simulink model "sym-project"  (R2023b)
settings: Solver=VariableStepAuto  StartTime=0.0  StopTime=5  RelTol=1e-3
undefined symbols (not defined in the file): A1_val, a1_val, A2_val, a2_val, A3_val, a3_val, A4_val, a4_val, A_numeric, B_numeric, C_numeric, g_val, K, k1, k1_val, k2_val, k_f, K_i, l_t, landa1_val, landa2_val
libraries: simulink x1
settings Model: Creator=Windows 10 2A-2017  LastModifiedBy=Asus
settings OptimizationCC: ReuseModelBlockBuffer=off

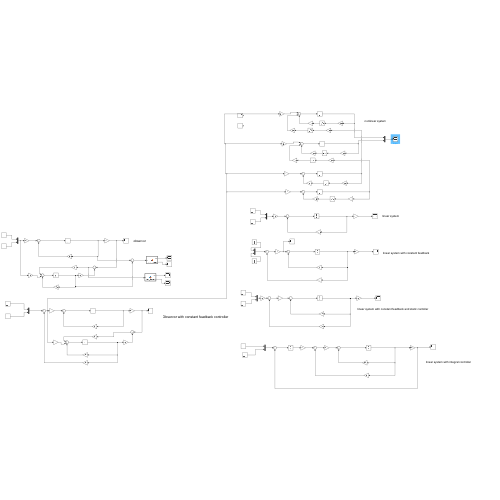
[thumbnail: Simulink's stored preview of the top-level diagram]
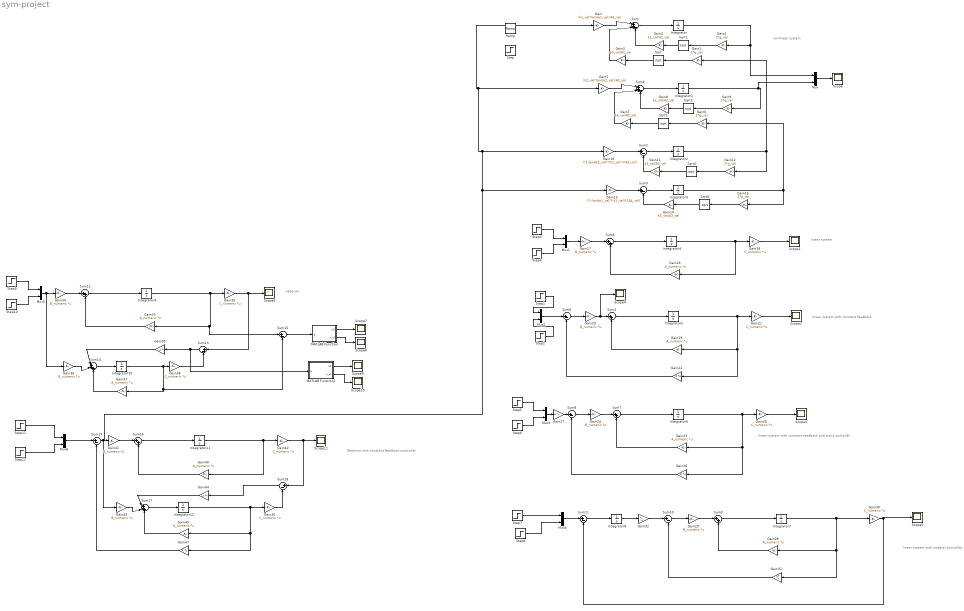
== system sym-project ==
  note: Observor with constant feadback controller
  note: linear system with constant feadback
  note: linear system
  note: nonlinear system
  note: linear system with constant feadback and static contoller
  note: linear system with integral controller
  note: observor
  Gain : Gain  Gain=(k1_val*landa1_val)/A1_val
  Gain{1,4,6,9,12,15} (6 alike) : Gain  Gain=2*g_val
  Gain10 : Gain  Gain=((1-landa2_val)*(k2_val))/(A3_val)
  Gain11 : Gain  Gain=a3_val/A3_val
  Gain13 : Gain  Gain=((1-landa1_val)*(k1_val))/(A4_val)
  Gain14 : Gain  Gain=a3_val/A3_val
  Gain{16,19,23,28,33,37,40,45} (8 alike) : Gain  Gain=A_numeric  Multiplication=Matrix(K*u)
  Gain{17,20,24,29,34,36,41,43} (8 alike) : Gain  Gain=B_numeric  Multiplication=Matrix(K*u)
  Gain{18,21,25,30,35,38,42,46} (8 alike) : Gain  Gain=C_numeric  Multiplication=Matrix(K*u)
  Gain2 : Gain  Gain=a3_val/A1_val
  Gain22 : Gain  Gain=K  Multiplication=Matrix(K*u)
  Gain26 : Gain  Gain=K  Multiplication=Matrix(K*u)
  Gain27 : Gain  Gain=k1  Multiplication=Matrix(K*u)
  Gain3 : Gain  Gain=a1_val/A1_val
  Gain31 : Gain  Gain=k_f  Multiplication=Matrix(K*u)
  Gain32 : Gain  Gain=K_i  Multiplication=Matrix(K*u)
  Gain39 : Gain  Gain=l_t  Multiplication=Matrix(K*u)
  Gain44 : Gain  Gain=l_t  Multiplication=Matrix(K*u)
  Gain47 : Gain  Gain=K  Multiplication=Matrix(K*u)
  Gain5 : Gain  Gain=(k2_val*landa2_val)/A2_val
  Gain7 : Gain  Gain=a4_val/A2_val
  Gain8 : Gain  Gain=a2_val/A2_val
  Integrator{,1..3} (4 alike) : Integrator
  Integrator{4,6,9..10,12} (5 alike) : Integrator  InitialCondition=[0;0;0;0]
  Integrator11 : Integrator  InitialCondition=[0.1;0.2;0.5;2]
  Integrator5 : Integrator  InitialCondition=[1;1.3;0.1;4]
  Integrator7 : Integrator  InitialCondition=[1,1.3,0.1,4]
  Integrator8 : Integrator  InitialCondition=[0.1;0.1]
  MATLAB Function : MATLAB Function  TreatAsAtomicUnit=on
  MATLAB Function1 : MATLAB Function  TreatAsAtomicUnit=on
  Mux{,1..6} (7 alike) : Mux  Inputs=2
  Ramp : simulink/Sources/Ramp  slope=1  start=0  InitialOutput=0
  Scope{,1..11} (12 alike) : Scope
  Sqrt{,1..5} (6 alike) : Sqrt
  Step{,3..6,9..10} (7 alike) : Step  Time=0  SampleTime=0
  Step{1..2,7..8,11..12} (6 alike) : Step  Time=0  After=0  SampleTime=0
  Sum : Sum  Inputs=|++-
  Sum1 : Sum  Inputs=|++-
  Sum{2..3,6,8,10..11,13,15,18..19} (10 alike) : Sum  Inputs=|+-
  Sum{4..5,7,9,12,16} (6 alike) : Sum  Inputs=|++
  Sum14 : Sum  Inputs=|+++
  Sum17 : Sum  Inputs=|+++
  wires:
  Gain/1 -> Sum/1
  Gain1/1 -> Sqrt/1
  Sqrt/1 -> Gain2/1
  Gain2/1 -> Sum/2
  Gain4/1 -> Sqrt1/1
  Sqrt1/1 -> Gain3/1
  Gain3/1 -> Sum/3
  Sum/1 -> Integrator/1
  Integrator/1 -> Mux/1, Gain4/1
  Gain8/1 -> Sum1/3
  Gain7/1 -> Sum1/2
  Sqrt3/1 -> Gain8/1
  Integrator1/1 -> Mux/2, Gain9/1
  Sum1/1 -> Integrator1/1
  Sqrt2/1 -> Gain7/1
  Gain5/1 -> Sum1/1
  Gain6/1 -> Sqrt2/1
  Gain9/1 -> Sqrt3/1
  Sqrt4/1 -> Gain11/1
  Gain12/1 -> Sqrt4/1
  Gain11/1 -> Sum2/2
  Sum2/1 -> Integrator2/1
  Gain10/1 -> Sum2/1
  Gain14/1 -> Sum3/2
  Gain15/1 -> Sqrt5/1
  Sqrt5/1 -> Gain14/1
  Sum3/1 -> Integrator3/1
  Integrator2/1 -> Gain1/1, Gain12/1
  Integrator3/1 -> Gain6/1, Gain15/1
  Gain13/1 -> Sum3/1
  Mux/1 -> Scope/1
  Sum5/1 -> Integrator4/1
  Gain16/1 -> Sum5/2
  Integrator4/1 -> Gain16/1, Gain18/1
  Gain17/1 -> Sum5/1
  Mux1/1 -> Gain17/1
  Step3/1 -> Mux1/1
  Step4/1 -> Mux1/2
  Gain18/1 -> Scope1/1
  Gain21/1 -> Scope2/1
  Integrator5/1 -> Gain22/1, Gain19/1, Gain21/1
  Step2/1 -> Mux2/2
  Step1/1 -> Mux2/1
  Gain19/1 -> Sum4/2
  Sum4/1 -> Integrator5/1
  Gain22/1 -> Sum6/2
  Sum6/1 -> Gain20/1
  Gain20/1 -> Scope4/1, Sum4/1
  Mux2/1 -> Sum6/1
  Sum8/1 -> Gain24/1
  Gain26/1 -> Sum8/2
  Integrator6/1 -> Gain26/1, Gain23/1, Gain25/1
  Step5/1 -> Mux3/1
  Gain23/1 -> Sum7/2
  Sum7/1 -> Integrator6/1
  Gain25/1 -> Scope3/1
  Step6/1 -> Mux3/2
  Gain24/1 -> Sum7/1
  Mux3/1 -> Gain27/1
  Gain27/1 -> Sum8/1
  Gain29/1 -> Sum9/1
  Gain31/1 -> Sum10/2
  Gain28/1 -> Sum9/2
  Integrator7/1 -> Gain31/1, Gain28/1, Gain30/1
  Sum10/1 -> Gain29/1
  Step8/1 -> Mux4/2
  Step7/1 -> Mux4/1
  Mux4/1 -> Sum11/1
  Sum11/1 -> Integrator8/1
  Integrator8/1 -> Gain32/1
  Gain32/1 -> Sum10/1
  Sum9/1 -> Integrator7/1
  Gain30/1 -> Sum11/2, Scope5/1
  Gain34/1 -> Sum12/1
  Sum12/1 -> Integrator9/1
  Gain35/1 -> Sum13/1, Scope6/1
  Step9/1 -> Mux5/1
  Mux5/1 -> Gain36/1, Gain34/1
  Gain33/1 -> Sum12/2
  Step10/1 -> Mux5/2
  Integrator9/1 -> Sum15/1, Gain33/1, Gain35/1
  Sum14/1 -> Integrator10/1
  Integrator10/1 -> Gain38/1, Sum15/2, Gain37/1
  Gain38/1 -> Sum13/2
  Sum13/1 -> MATLAB Function1/1(e), Gain39/1
  Gain37/1 -> Sum14/3
  Gain36/1 -> Sum14/2
  Gain39/1 -> Sum14/1
  Sum15/1 -> MATLAB Function/1(e)
  MATLAB Function/1(n2) -> Scope7/1
  MATLAB Function/2(ninf) -> Scope8/1
  MATLAB Function1/1(n2) -> Scope9/1
  MATLAB Function1/2(ninf) -> Scope10/1
  Integrator11/1 -> Gain40/1, Gain42/1
  Sum16/1 -> Integrator11/1
  Step11/1 -> Mux6/1
  Gain41/1 -> Sum16/1
  Gain42/1 -> Sum18/1, Scope11/1
  Gain40/1 -> Sum16/2
  Step12/1 -> Mux6/2
  Gain44/1 -> Sum17/1
  Gain43/1 -> Sum17/2
  Sum17/1 -> Integrator12/1
  Gain45/1 -> Sum17/3
  Integrator12/1 -> Gain46/1, Gain45/1, Gain47/1
  Sum18/1 -> Gain44/1
  Gain46/1 -> Sum18/2
  Mux6/1 -> Sum19/1
  Sum19/1 -> Gain/1, Gain5/1, Gain10/1, Gain13/1, Gain43/1, Gain41/1
  Gain47/1 -> Sum19/2

== matlab function sym-project/MATLAB Function ==
  data: e input; n2 output; ninf output
function [n2, ninf] = calc_norms(e)
n2   = sqrt(sum(e.^2));   
ninf = max(abs(e));       
end

== matlab function sym-project/MATLAB Function1 ==
  data: e input; n2 output; ninf output
function [n2, ninf] = calc_norms(e)
n2   = sqrt(sum(e.^2));   
ninf = max(abs(e));       
end
